simulink model "DynKepler"  (R2018b)
settings: configuration reference "Configuration" (kept outside this file)
model workspace (MATLAB code in the model file):
  | CON = Simulink.Parameter;
  | CON.DataType = 'Bus: Bus_CON';
  | CON.Value = Simulink.Bus.createMATLABStruct('Bus_CON');
settings Model: ParameterArgumentNames=CON  OrderedModelArguments=off  Creator=Ethan  LastModifiedBy=Ethan
settings ConfigSetRef: SourceLocation=Base Workspace

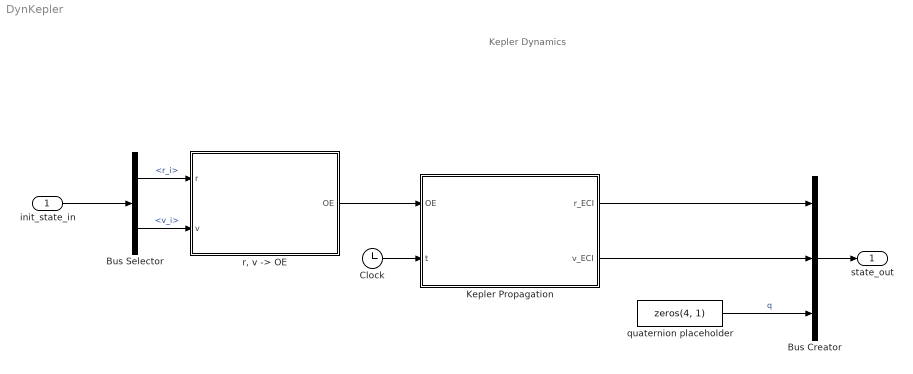
== system DynKepler ==
  note: Kepler Dynamics
  init_state_in : Inport  OutDataTypeStr=Bus: Bus_state
  Bus Creator : BusCreator  Inputs=3  OutDataTypeStr=Bus: Bus_state  NonVirtualBus=on
      settings: InheritFromInputs=off
  Bus Selector : BusSelector  OutputSignals=r_i,v_i
  Clock : Clock
  Kepler Propagation : MATLAB Function  TreatAsAtomicUnit=on
  quaternion placeholder : Constant  Value=zeros(4, 1)
  "r, v -> OE" : MATLAB Function  TreatAsAtomicUnit=on
  state_out : Outport  OutDataTypeStr=Bus: Bus_state
  wires:
  init_state_in/1 -> Bus Selector/1
  quaternion placeholder/1 -> Bus Creator/3  "q"
  Bus Creator/1 -> state_out/1
  Bus Selector/1 -> "r, v -> OE"/1(r)  "<r_i>"
  Bus Selector/2 -> "r, v -> OE"/2(v)  "<v_i>"
  "r, v -> OE"/1(OE) -> Kepler Propagation/1(OE)
  Kepler Propagation/2(v_ECI) -> Bus Creator/2
  Kepler Propagation/1(r_ECI) -> Bus Creator/1
  Clock/1 -> Kepler Propagation/2(t)

== matlab function DynKepler/Kepler Propagation ==
  data: OE input; r_ECI output; t input; CON parameter; v_ECI output
function [r_ECI, v_ECI] = kepler_prop(OE, t, CON)
a = OE.a;
e = OE.e;
inc = OE.inc;
omega = OE.omega;
w = OE.w;
nu = OE.nu;

persistent t0 E0 M0 n
if isempty(t0)
    t0 = t;
    E0 = 2 * atan(sqrt((1 - e) / (1 + e)) * tand(nu / 2));
    M0 = E0 - e * sin(E0);
    n = sqrt(CON.mu / a ^ 3);
end

M = mod(M0 + n * (t - t0), 2 * pi);
E = M2E(M,e,1e-8);
nu_prop = 2 * atand(sqrt((1 + e) / (1 - e)) * tan(E / 2));

[r_ECI,v_ECI] = oe2rvECI(a,e,inc,omega,w,nu_prop);

end

== matlab function DynKepler/r, v -> OE ==
  data: r input; v input; OE output Bus: Bus_OE; CON parameter
function OE = pos2oe(r, v, CON)

[OE.a,OE.e,OE.inc,OE.omega,OE.w,OE.nu] = rvECI2oe(r,v,CON.mu);
